simulink model "spiBitbangSimulink_v4"  (R2013b)
settings: Solver=ode3  StartTime=0.0  StopTime=5e-3  FixedStep=sampleTime  MaxStep=MaxStepSize  RelTol=1e-3
undefined symbols (not defined in the file or in its folder): High, Low, periSam, pulseSam, sampleTime
libraries: dspswit3 x9, simulink x4
settings Model: ExtModeTrigDuration=100  Creator=mainster  LastModifiedBy=mainster
settings OptimizationCC: OptimizeModelRefInitCode=on  LifeSpan=1
settings DebuggingCC: SolverPrmCheckMsg=none
settings HardwareCC: ProdLargestAtomicInteger=Long  ProdLargestAtomicFloat=Double  ProdEndianess=LittleEndian  ProdHWDeviceType=ARM Compatible->ARM Cortex
settings RTWCC: SystemTargetFile=realtime.tlc  GenerateMakefile=off  TemplateMakefile=realtime.tmf  Description=Run on Target Hardware  RTWVerbose=off  ProcessScript=realtime_make_rtw_hook
settings STFCustomTargetCC: TargetLibSuffix=.a  GenerateSampleERTMain=on  ERTCustomFileBanners=on  SupportNonInlinedSFcns=off  SupportVariableSizeSignals=on  MATLABClassNameForMDSCustomization=Simulink.SoftwareTarget.ERTCustomization  GRTInterface=off  SystemTargetFile=realtime.tlc
settings ERTTargetCC: CodeReplacementLibrary=ANSI_C  GenerateSampleERTMain=on  ParMdlRefBuildCompliant=off  CompOptLevelCompliant=off  ConcurrentExecutionCompliant=off  CombineOutputUpdateFcns=off  ERTFirstTimeCompliant=off  SupportContinuousTime=on  SupportVariableSizeSignals=on  ModelStepFunctionPrototypeControlCompliant=off  CPPClassGenCompliant=off  ExtModeMexArgs='192.168.2.111' 0 17725  InlinedParameterPlacement=NonHierarchical  ERTSrcFileBannerTemplate=realtime_code_template.cgt  ERTHdrFileBannerTemplate=realtime_code_template.cgt  ERTDataSrcFileTemplate=realtime_code_template.cgt  ERTDataHdrFileTemplate=realtime_code_template.cgt  ERTCustomFileTemplate=realtime_file_process.tlc

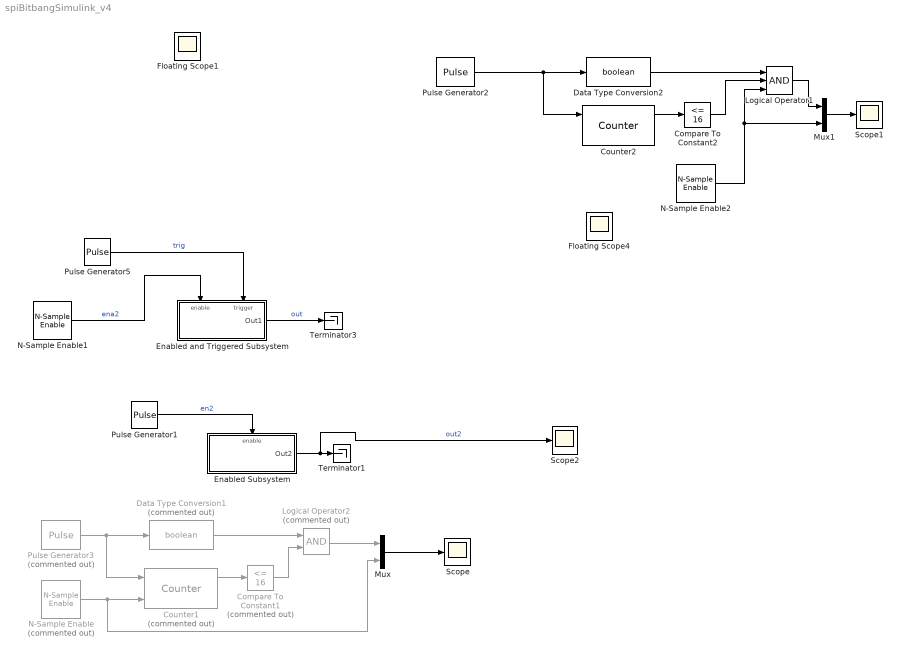
== system spiBitbangSimulink_v4 ==
  Compare To Constant1 : simulink/Logic and Bit Operations/Compare To Constant  Commented=on  relop=<=  const=16  OutDataTypeStr=boolean
  Compare To Constant2 : simulink/Logic and Bit Operations/Compare To Constant  relop=<=  const=16  OutDataTypeStr=boolean
  Counter1 : dspswit3/Counter  Commented=on  Direction=Down  CountEvent=Rising edge  CounterSize=User defined  MaxCount=20  InitialCount=0  Output=Count and Hit  HitValue=4  ResetInput=on  SamplesPerFrame=1  Ts=1  CntDtype=double  HitDtype=Logical
  Counter2 : dspswit3/Counter  Direction=Down  CountEvent=Rising edge  CounterSize=User defined  MaxCount=20  InitialCount=0  Output=Count and Hit  HitValue=4  ResetInput=on  SamplesPerFrame=1  Ts=1  CntDtype=double  HitDtype=Logical
  Data Type Conversion1 : DataTypeConversion  Commented=on  OutDataTypeStr=boolean
  Data Type Conversion2 : DataTypeConversion  OutDataTypeStr=boolean
  Enabled Subsystem : Subsystem  TreatAsAtomicUnit=on
  Enabled and Triggered Subsystem : Subsystem  TreatAsAtomicUnit=on
  Floating Scope4 : Scope  NumInputPorts=3
      settings: Floating=on  TimeRange=0.005  YMin=-0.1~-0.1~-0.1  YMax=1.1~1.1~1.1  SaveName=ScopeData5
  Logical Operator1 : Logic  Inputs=3  AllPortsSameDT=off  OutDataTypeStr=boolean
  Logical Operator2 : Logic  Commented=on  AllPortsSameDT=off  OutDataTypeStr=boolean
  Mux : Mux  Inputs=2
  Mux1 : Mux  Inputs=2
  N-Sample Enable : dspswit3/N-Sample Enable  Commented=on  N=250  ActiveLevel=High (1)  reset=off  TriggerType=Rising edge  Ts=sampleTime  DataType=Logical
  N-Sample Enable1 : dspswit3/N-Sample Enable  N=250  ActiveLevel=High (1)  reset=off  TriggerType=Rising edge  Ts=sampleTime  DataType=Logical
  N-Sample Enable2 : dspswit3/N-Sample Enable  N=16*periSam  ActiveLevel=Low (0)  reset=off  TriggerType=Rising edge  Ts=-1  DataType=Logical
  Pulse Generator1 : DiscretePulseGenerator  Period=800  PulseWidth=700  SampleTime=-1
  Pulse Generator2 : DiscretePulseGenerator  Period=periSam  PulseWidth=pulseSam  SampleTime=-1
  Pulse Generator3 : DiscretePulseGenerator  Commented=on  Period=50  PulseWidth=25  SampleTime=sampleTime
  Pulse Generator5 : DiscretePulseGenerator  Period=200  PulseWidth=150  SampleTime=-1
  Scope : Scope
      settings: SaveName=ScopeData2
  Scope1 : Scope
      settings: TimeRange=0.005  YMin=-0.1  YMax=1.1
  Scope2 : Scope
      settings: TimeRange=0.005  YMin=-0.1  YMax=1.1
  Terminator1 : Terminator
  Terminator3 : Terminator
  Floating Scope1 : Scope
      settings: Floating=on  SaveName=ScopeData3
  wires:
  Pulse Generator3/1 -> Counter1/1, Data Type Conversion1/1
  N-Sample Enable/1 -> Counter1/2, Mux/2
  Data Type Conversion1/1 -> Logical Operator2/1
  Logical Operator2/1 -> Mux/1
  Mux/1 -> Scope/1
  Counter1/1 -> Compare To Constant1/1
  Compare To Constant1/1 -> Logical Operator2/2
  Enabled and Triggered Subsystem/1(Out1) -> Terminator3/1  "out"
  Pulse Generator5/1 -> Enabled and Triggered Subsystem/Trigger  "trig"
  N-Sample Enable1/1 -> Enabled and Triggered Subsystem/Enable  "ena2"
  Enabled Subsystem/1(Out2) -> Scope2/1, Terminator1/1  "out2"
  Pulse Generator1/1 -> Enabled Subsystem/Enable  "en2"
  Pulse Generator2/1 -> Counter2/1, Data Type Conversion2/1
  Data Type Conversion2/1 -> Logical Operator1/1
  Counter2/1 -> Compare To Constant2/1
  Compare To Constant2/1 -> Logical Operator1/2
  N-Sample Enable2/1 -> Mux1/2, Logical Operator1/3
  Mux1/1 -> Scope1/1
  Logical Operator1/1 -> Mux1/1

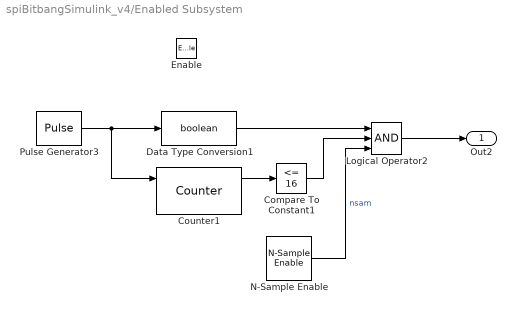
== system spiBitbangSimulink_v4/Enabled Subsystem ==
  Enable : EnablePort  StatesWhenEnabling=reset
  Compare To Constant1 : simulink/Logic and Bit Operations/Compare To Constant  relop=<=  const=16  OutDataTypeStr=boolean
  Counter1 : dspswit3/Counter  Direction=Down  CountEvent=Rising edge  CounterSize=User defined  MaxCount=16  InitialCount=0  Output=Count and Hit  HitValue=4  ResetInput=on  SamplesPerFrame=1  Ts=1  CntDtype=double  HitDtype=Logical
  Data Type Conversion1 : DataTypeConversion  OutDataTypeStr=boolean
  Logical Operator2 : Logic  Inputs=3  AllPortsSameDT=off  OutDataTypeStr=boolean
  N-Sample Enable : dspswit3/N-Sample Enable  N=16*periSam  ActiveLevel=Low (0)  reset=off  TriggerType=Rising edge  Ts=-1  DataType=Logical
  Pulse Generator3 : DiscretePulseGenerator  Period=periSam  PulseWidth=pulseSam  SampleTime=-1
  Out2 : Outport
  wires:
  Pulse Generator3/1 -> Counter1/1, Data Type Conversion1/1
  Data Type Conversion1/1 -> Logical Operator2/1
  Counter1/1 -> Compare To Constant1/1
  Compare To Constant1/1 -> Logical Operator2/2
  Logical Operator2/1 -> Out2/1
  N-Sample Enable/1 -> Logical Operator2/3  "nsam"

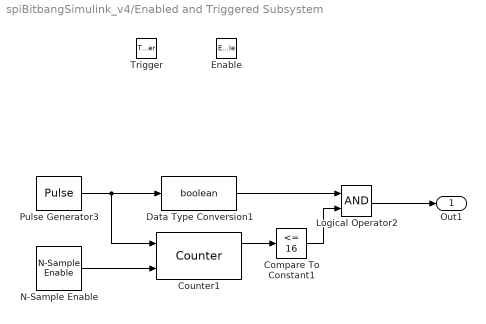
== system spiBitbangSimulink_v4/Enabled and Triggered Subsystem ==
  Enable : EnablePort
  Trigger : TriggerPort
  Compare To Constant1 : simulink/Logic and Bit Operations/Compare To Constant  relop=<=  const=16  OutDataTypeStr=boolean
  Counter1 : dspswit3/Counter  Direction=Down  CountEvent=Rising edge  CounterSize=User defined  MaxCount=20  InitialCount=0  Output=Count and Hit  HitValue=4  ResetInput=on  SamplesPerFrame=1  Ts=1  CntDtype=double  HitDtype=Logical
  Data Type Conversion1 : DataTypeConversion  OutDataTypeStr=boolean
  Logical Operator2 : Logic  AllPortsSameDT=off  OutDataTypeStr=boolean
  N-Sample Enable : dspswit3/N-Sample Enable  N=250  ActiveLevel=High (1)  reset=off  TriggerType=Rising edge  Ts=-1  DataType=Logical
  Pulse Generator3 : DiscretePulseGenerator  Period=50  PulseWidth=25  SampleTime=-1
  Out1 : Outport
  wires:
  Pulse Generator3/1 -> Counter1/1, Data Type Conversion1/1
  N-Sample Enable/1 -> Counter1/2
  Data Type Conversion1/1 -> Logical Operator2/1
  Counter1/1 -> Compare To Constant1/1
  Compare To Constant1/1 -> Logical Operator2/2
  Logical Operator2/1 -> Out1/1
